simulink model "DC_Motor_Velocity_Control_Archieve"  (R2018b)
settings: Solver=VariableStepAuto  StartTime=0.0  StopTime=10.0  RelTol=1e-3
values from neighbouring files (symbols this model uses):
  b = 22.5    [DC_Simulink.m]
  J = 2.21E-6    (= 2.21e-06)    [DC_Servomotor_Code.m]    (also in DC_Simulink.m = 0.306)
  K = 0.055    [DC_Servomotor_Code.m]    (also in DC_Simulink.m = 0.109)
  L = 5.02E-3    (= 0.00502)    [DC_Servomotor_Code.m]    (also in DC_Simulink.m = 0.000625)
  R = 41.5    [DC_Servomotor_Code.m]    (also in DC_Simulink.m = 0.522)
  Tload = TL(1,i)    [DC_Simulink.m]
libraries: simulink x3, fuzblock x1
settings Model: Creator=james.quan.166  LastModifiedBy=james.quan.166

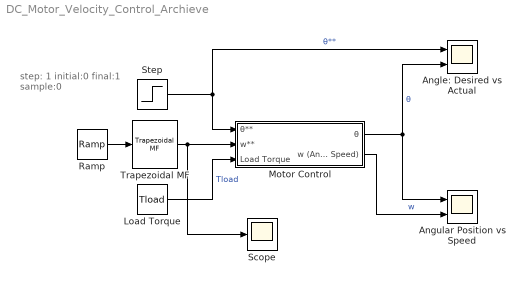
== system DC_Motor_Velocity_Control_Archieve ==
  note: step: 1
      | initial:0
      | final:1
      | sample:0
  Angle: Desired vs Actual : Scope  NumInputPorts=2
  Angular Position vs Speed : Scope  NumInputPorts=2
  Load Torque : Constant  Value=Tload
  Motor Control : Subsystem
  Ramp : simulink/Sources/Ramp  slope=2  start=0  InitialOutput=0
  Scope : Scope
  Step : Step  SampleTime=0
  Trapezoidal MF : fuzblock/Membership  Functions/Trapezoidal MF  a=0  b=1  c=1  d=2
      settings: SourceProductName=Fuzzy Logic Toolbox  SourceProductBaseCode=FL
  wires:
  Trapezoidal MF/1 -> Scope/1, Motor Control/2(w**)
  Load Torque/1 -> Motor Control/3(Load Torque)  "Tload"
  Motor Control/2(w (Angular Speed)) -> Angular Position vs Speed/2  "w"
  Step/1 -> Motor Control/1(θ**), Angle: Desired vs Actual/1  "θ**"
  Motor Control/1(θ) -> Angle: Desired vs Actual/2, Angular Position vs Speed/1  "θ"
  Ramp/1 -> Trapezoidal MF/1

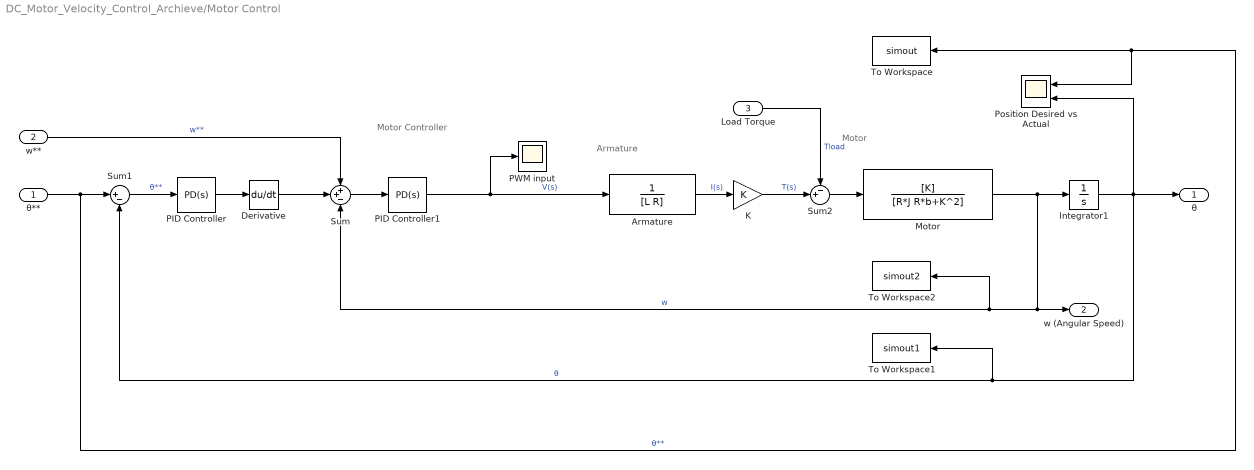
== system DC_Motor_Velocity_Control_Archieve/Motor Control ==
  note: Armature
  note: Motor
  note: Motor Controller
  θ** : Inport
  w** : Inport  Port=2
  Load Torque : Inport  Port=3
  Armature : TransferFcn  Denominator=[L R]
  Derivative : Derivative
  Integrator1 : Integrator
  K : Gain  Gain=K
  Motor : TransferFcn  Numerator=[K]  Denominator=[R*J R*b+K^2]
  PID Controller : simulink/Continuous/PID Controller  Controller=PD  Form=Parallel  TimeDomain=Continuous-time  SampleTime=-1  IntegratorMethod=Forward Euler  FilterMethod=Forward Euler  ControllerParametersSource=internal  P=1  I=648207.462988784  D=0  UseFilter=on  N=100  TunerSelectOption=Transfer Function Based (PID Tuner App)  InitialConditionSource=internal  InitialConditionForIntegrator=0  InitialConditionForFilter=0  DifferentiatorICPrevScaledInput=0  ExternalReset=none  TrackingMode=off  Kt=1  LimitOutput=off  UpperSaturationLimit=inf  LowerSaturationLimit=-inf  LinearizeAsGain=on  AntiWindupMode=none  Kb=1  POutMin=[]  POutMax=[]  IOutMin=[]  IOutMax=[]  DOutMin=[]  DOutMax=[]  NOutMin=[]  NOutMax=[]  SumOutMin=[]  SumOutMax=[]  SaturationOutMin=[]  SaturationOutMax=[]  PParamMin=[]  PParamMax=[]  IParamMin=[]  IParamMax=[]  DParamMin=[]  DParamMax=[]  NParamMin=[]  NParamMax=[]  KbParamMin=[]  KbParamMax=[]  KtParamMin=[]  KtParamMax=[]  KbOutMin=[]  KbOutMax=[]  KtOutMin=[]  KtOutMax=[]  IntegratorOutMin=[]  IntegratorOutMax=[]  FilterOutMin=[]  FilterOutMax=[]  SumI1OutMin=[]  SumI1OutMax=[]  SumI2OutMin=[]  SumI2OutMax=[]  SumI3OutMin=[]  SumI3OutMax=[]  SumI4OutMin=[]  SumI4OutMax=[]  SumDOutMin=[]  SumDOutMax=[]  DifferentiatorOutMin=[]  DifferentiatorOutMax=[]  FilterDiffOutCoefMin=[]  FilterDiffOutCoefMax=[]  ReciprocalOutMin=[]  ReciprocalOutMax=[]  SumDenOutMin=[]  SumDenOutMax=[]  SumNumOutMin=[]  SumNumOutMax=[]  DivideOutMin=[]  DivideOutMax=[]  IntegratorContinuousStateAttributes=''  IntegratorStateMustResolveToSignalObject=off  IntegratorRTWStateStorageClass=Auto  FilterContinuousStateAttributes=''  FilterStateMustResolveToSignalObject=off  FilterRTWStateStorageClass=Auto  ParallelPVariant=InternalParameters  IdealPVariant=Disabled  IVariant=Disabled  DVariant=InternalParameters  IntegratorVariant=Disabled  SatVariant=Disabled  AWVariant=Disabled  PCopyVariant=Disabled  TRVariant=Disabled  FdbkBlocksVariant=Forward  IdealPFdbkVariant=Disabled  SatFdbkVariant=Disabled  DerivativeFilterVariant=ContFilter  NVariant=InternalParameters  NCopyVariant=Disabled  FilterICVariant=InternalICsFilter  IntegratorICVariant=Disabled  ExternalResetVariant=Disabled  TRSumVariant=Passthrough  SumFdbkVariant=Disabled  SumVariant=Sum_PD
  PID Controller1 : simulink/Continuous/PID Controller  Controller=PD  Form=Parallel  TimeDomain=Continuous-time  SampleTime=-1  IntegratorMethod=Forward Euler  FilterMethod=Forward Euler  ControllerParametersSource=internal  P=15804662796.2051  I=648207.462988784  D=27543.6313433708  UseFilter=on  N=82076025.2592576  TunerSelectOption=Transfer Function Based (PID Tuner App)  InitialConditionSource=internal  InitialConditionForIntegrator=0  InitialConditionForFilter=0  DifferentiatorICPrevScaledInput=0  ExternalReset=none  TrackingMode=off  Kt=1  LimitOutput=off  UpperSaturationLimit=inf  LowerSaturationLimit=-inf  LinearizeAsGain=on  AntiWindupMode=none  Kb=1  POutMin=[]  POutMax=[]  IOutMin=[]  IOutMax=[]  DOutMin=[]  DOutMax=[]  NOutMin=[]  NOutMax=[]  SumOutMin=[]  SumOutMax=[]  SaturationOutMin=[]  SaturationOutMax=[]  PParamMin=[]  PParamMax=[]  IParamMin=[]  IParamMax=[]  DParamMin=[]  DParamMax=[]  NParamMin=[]  NParamMax=[]  KbParamMin=[]  KbParamMax=[]  KtParamMin=[]  KtParamMax=[]  KbOutMin=[]  KbOutMax=[]  KtOutMin=[]  KtOutMax=[]  IntegratorOutMin=[]  IntegratorOutMax=[]  FilterOutMin=[]  FilterOutMax=[]  SumI1OutMin=[]  SumI1OutMax=[]  SumI2OutMin=[]  SumI2OutMax=[]  SumI3OutMin=[]  SumI3OutMax=[]  SumI4OutMin=[]  SumI4OutMax=[]  SumDOutMin=[]  SumDOutMax=[]  DifferentiatorOutMin=[]  DifferentiatorOutMax=[]  FilterDiffOutCoefMin=[]  FilterDiffOutCoefMax=[]  ReciprocalOutMin=[]  ReciprocalOutMax=[]  SumDenOutMin=[]  SumDenOutMax=[]  SumNumOutMin=[]  SumNumOutMax=[]  DivideOutMin=[]  DivideOutMax=[]  IntegratorContinuousStateAttributes=''  IntegratorStateMustResolveToSignalObject=off  IntegratorRTWStateStorageClass=Auto  FilterContinuousStateAttributes=''  FilterStateMustResolveToSignalObject=off  FilterRTWStateStorageClass=Auto  ParallelPVariant=InternalParameters  IdealPVariant=Disabled  IVariant=Disabled  DVariant=InternalParameters  IntegratorVariant=Disabled  SatVariant=Disabled  AWVariant=Disabled  PCopyVariant=Disabled  TRVariant=Disabled  FdbkBlocksVariant=Forward  IdealPFdbkVariant=Disabled  SatFdbkVariant=Disabled  DerivativeFilterVariant=ContFilter  NVariant=InternalParameters  NCopyVariant=Disabled  FilterICVariant=InternalICsFilter  IntegratorICVariant=Disabled  ExternalResetVariant=Disabled  TRSumVariant=Passthrough  SumFdbkVariant=Disabled  SumVariant=Sum_PD
  PWM input : Scope
  Position Desired vs Actual : Scope  NumInputPorts=2
  Sum : Sum  Inputs=++-
  Sum1 : Sum  Inputs=|+-
  Sum2 : Sum  Inputs=-+|
  To Workspace : ToWorkspace  VariableName=simout  SaveFormat=Timeseries  SampleTime=-1
  To Workspace1 : ToWorkspace  VariableName=simout1  SaveFormat=Timeseries  SampleTime=-1
  To Workspace2 : ToWorkspace  VariableName=simout2  SaveFormat=Timeseries  SampleTime=-1
  θ : Outport
  w (Angular Speed) : Outport  Port=2
  wires:
  Motor/1 -> w (Angular Speed)/1, To Workspace2/1, Sum/3, Integrator1/1  "w"
  K/1 -> Sum2/2  "T(s)"
  PID Controller/1 -> Derivative/1
  Sum2/1 -> Motor/1
  Load Torque/1 -> Sum2/1  "Tload"
  Integrator1/1 -> θ/1, To Workspace1/1, Sum1/2, Position Desired vs Actual/2  "θ"
  Sum1/1 -> PID Controller/1  "θ**"
  θ**/1 -> To Workspace/1, Position Desired vs Actual/1, Sum1/1  "θ**"
  Armature/1 -> K/1  "I(s)"
  PID Controller1/1 -> PWM input/1, Armature/1  "V(s)"
  Sum/1 -> PID Controller1/1
  w**/1 -> Sum/1  "w**"
  Derivative/1 -> Sum/2
